simulink library "Damper_LeftRight_Nonlinear"  (R2025b)
settings: Solver=VariableStepAuto  StartTime=0.0  StopTime=10.0  RelTol=1e-3
libraries: Damper_Nonlinear x2, fl_lib x2
Description:
  | Component of Simscape Vehicle Templates Library
  | 
  | Copyright 2018-2025 The MathWorks, Inc.
settings Model: Creator=smiller  LastModifiedBy=smiller
settings SolverCC: AlgebraicLoopSolver=TrustRegion
settings DataIOCC: ReturnWorkspaceOutputs=off
settings OptimizationCC: ReuseModelBlockBuffer=off
settings DebuggingCC: UnconnectedInputMsg=warning  UnconnectedOutputMsg=warning  UnconnectedLineMsg=warning  ArithmeticOperatorsInVariantConditions=warning
settings ModelReferenceCC: EnableRefExpFcnMdlSchedulingChecks=on
settings SFSimCC: CustomCodeUndefinedFunction=UseInterfaceOnly
settings RTWCC: GPUComputeCapability=3.5  DLArmComputeVersion=19.05

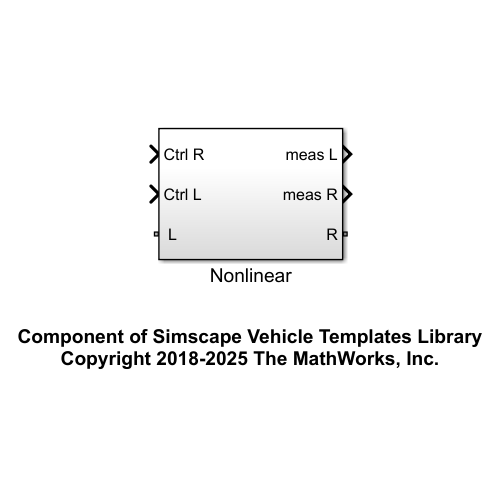
[thumbnail: Simulink's stored preview of the top-level diagram]
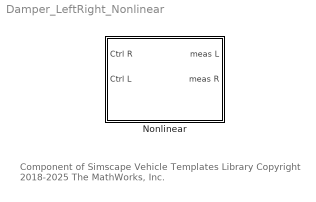
== system Damper_LeftRight_Nonlinear ==
  note: Component of Simscape Vehicle Templates Library
      | Copyright 2018-2025 The MathWorks, Inc.
  Nonlinear : Subsystem  VariantControl=Nonlinear

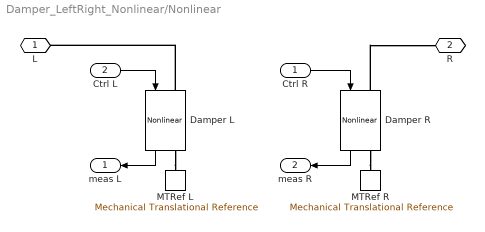
== system Damper_LeftRight_Nonlinear/Nonlinear ==
  Ctrl R : Inport
  Ctrl L : Inport  Port=2
  Damper L : Damper_Nonlinear/Nonlinear  VariantControl=Nonlinear  velocity_vector=Damper.Damping.vDamper.Value  force_vector=Damper.Damping.fDamper.Value  hp_dpr_top=Damper.Damping.sTop.Value  hp_dpr_bot=Damper.Damping.sBottom.Value  bs_lim_upper=Damper.Endstop.xMax.Value  bs_lim_lower=Damper.Endstop.xMin.Value  bs_k_upper=Damper.Endstop.KxMax.Value  bs_k_lower=Damper.Endstop.KxMin.Value  bs_b_upper=Damper.Endstop.dxMax.Value  bs_b_lower=Damper.Endstop.dxMin.Value  bs_region=Damper.Endstop.xTransition.Value
  Damper R : Damper_Nonlinear/Nonlinear  VariantControl=Nonlinear  velocity_vector=Damper.Damping.vDamper.Value  force_vector=Damper.Damping.fDamper.Value  hp_dpr_top=Damper.Damping.sTop.Value  hp_dpr_bot=Damper.Damping.sBottom.Value  bs_lim_upper=Damper.Endstop.xMax.Value  bs_lim_lower=Damper.Endstop.xMin.Value  bs_k_upper=Damper.Endstop.KxMax.Value  bs_k_lower=Damper.Endstop.KxMin.Value  bs_b_upper=Damper.Endstop.dxMax.Value  bs_b_lower=Damper.Endstop.dxMin.Value  bs_region=Damper.Endstop.xTransition.Value
  MTRef L : fl_lib/Mechanical/Translational Elements/Mechanical Translational Reference
  MTRef R : fl_lib/Mechanical/Translational Elements/Mechanical Translational Reference
  " L" : PMIOPort  Side=Left
  " R" : PMIOPort  Port=2  Side=Right
  meas L : Outport  VectorParamsAs1DForOutWhenUnconnected=off
  meas R : Outport  Port=2  VectorParamsAs1DForOutWhenUnconnected=off
  wires:
  Damper R/1 -> meas R/1
  Ctrl R/1 -> Damper R/1
  Ctrl L/1 -> Damper L/1
  Damper L/1 -> meas L/1
  connections:
  Damper L/LConn1 -- " L"/RConn1
  Damper R/RConn1 -- MTRef R/LConn1
  Damper R/LConn1 -- " R"/RConn1
  Damper L/RConn1 -- MTRef L/LConn1
